simulink model "power_systerm_model"  (R2025b)
settings: Solver=FixedStepDiscrete  StartTime=0.0  StopTime=10.0  FixedStep=0.005  RelTol=1e-3
values from neighbouring files (symbols this model uses):
  motorMaxReactionTorque_Nm = 0.055562    [PowerSystemDict.sldd]
  motorMaxThrust_N = 4.17944622    [PowerSystemDict.sldd]
  motorTimeConstant_s = 0.005    [PowerSystemDict.sldd]
undefined symbols (not defined in the file or in its folder): motorArmLength_m, Thrust_Body, Torque_Body
settings Model: DataDictionary=PowerSystemDict.sldd  Creator=89447  LastModifiedBy=89447

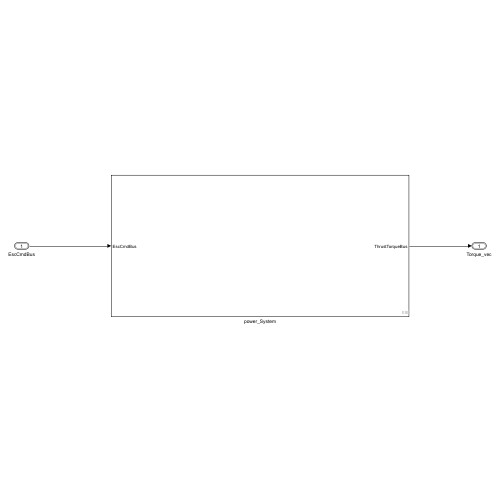
[thumbnail: Simulink's stored preview of the top-level diagram]
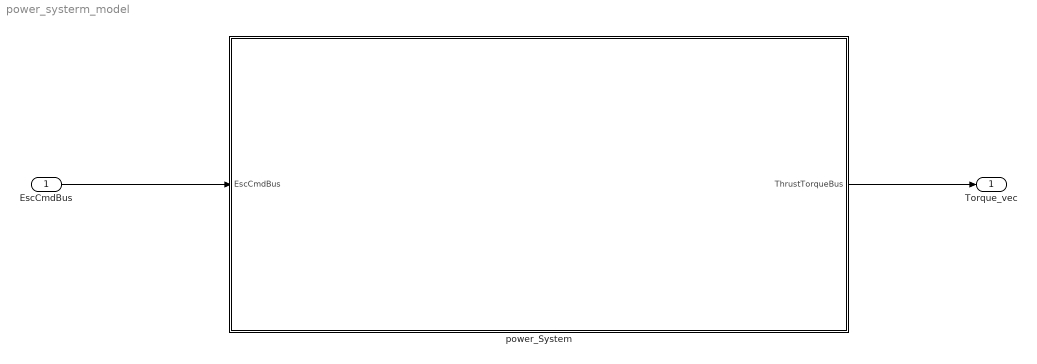
== system power_systerm_model ==
  EscCmdBus : Inport  OutDataTypeStr=Bus: EscCmdBus  LockScale=on  BusOutputAsStruct=on
  power_System : Subsystem
  Torque_vec : Outport  OutDataTypeStr=Bus: ThrustTorqueBus  LockScale=on  BusOutputAsStruct=on
  wires:
  EscCmdBus/1 -> power_System/1(EscCmdBus)
  power_System/1(ThrustTorqueBus) -> Torque_vec/1

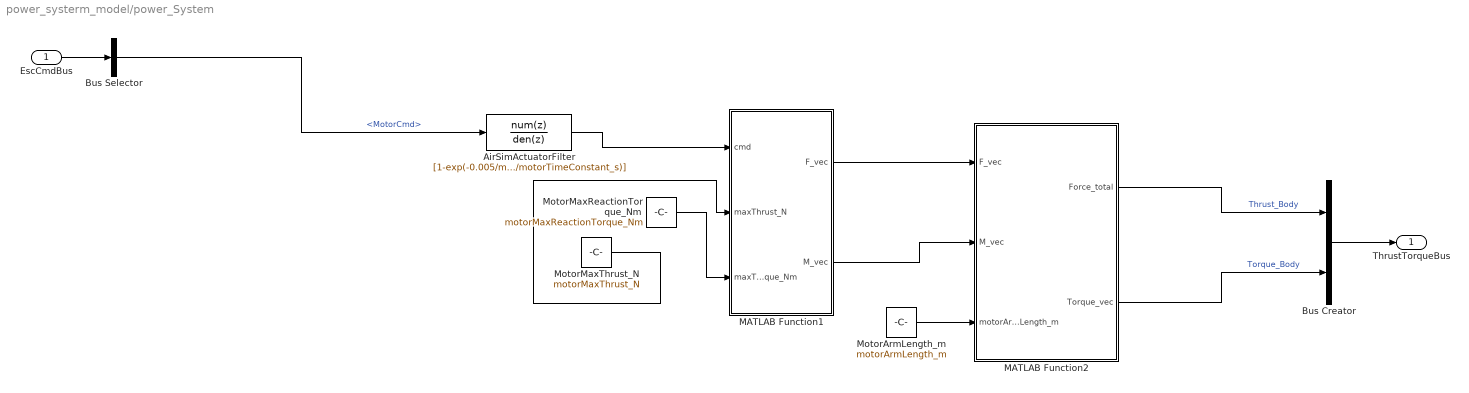
== system power_systerm_model/power_System ==
  EscCmdBus : Inport  OutDataTypeStr=Bus: EscCmdBus
  AirSimActuatorFilter : DiscreteTransferFcn  Numerator=[1-exp(-0.005/motorTimeConstant_s)]  Denominator=[1 -exp(-0.005/motorTimeConstant_s)]  SampleTime=0.005
  Bus Creator : BusCreator  Inputs=Thrust_Body,Torque_Body  OutDataTypeStr=Bus: ThrustTorqueBus
  Bus Selector : BusSelector  OutputSignals=MotorCmd
  MATLAB Function1 : MATLAB Function  TreatAsAtomicUnit=on
  MATLAB Function2 : MATLAB Function  TreatAsAtomicUnit=on
  MotorArmLength_m : Constant  Value=motorArmLength_m
  MotorMaxReactionTorque_Nm : Constant  Value=motorMaxReactionTorque_Nm
  MotorMaxThrust_N : Constant  Value=motorMaxThrust_N
  ThrustTorqueBus : Outport
  wires:
  MATLAB Function1/2(M_vec) -> MATLAB Function2/2(M_vec)
  MotorMaxReactionTorque_Nm/1 -> MATLAB Function1/3(maxTorque_Nm)
  MotorMaxThrust_N/1 -> MATLAB Function1/2(maxThrust_N)
  AirSimActuatorFilter/1 -> MATLAB Function1/1(cmd)
  MATLAB Function1/1(F_vec) -> MATLAB Function2/1(F_vec)
  MATLAB Function2/2(Torque_vec) -> Bus Creator/2  "Torque_Body"
  MotorArmLength_m/1 -> MATLAB Function2/3(motorArmLength_m)
  MATLAB Function2/1(Force_total) -> Bus Creator/1  "Thrust_Body"
  EscCmdBus/1 -> Bus Selector/1
  Bus Creator/1 -> ThrustTorqueBus/1
  Bus Selector/1 -> AirSimActuatorFilter/1  "<MotorCmd>"

== matlab function power_systerm_model/power_System/MATLAB Function1 ==
  data: cmd input; F_vec output; maxThrust_N input; maxTorque_Nm input; M_vec output
function [F_vec, M_vec] = fcn_airsim_rotors(cmd, maxThrust_N, maxTorque_Nm)
% AirSim RotorActuator: normalized command maps linearly to thrust and reaction torque.
cmd = max(single(0), min(single(1), single(cmd)));
F_vec = single(maxThrust_N) .* cmd;
M_vec = single(maxTorque_Nm) .* cmd;
end

== matlab function power_systerm_model/power_System/MATLAB Function2 ==
  data: F_vec input; Force_total output; M_vec input; motorArmLength_m input; Torque_vec output
function [Force_total, Torque_vec] = fcn_geometry_mixer(F_vec, M_vec, motorArmLength_m)
% AirSim QuadX rotor order and controller mixer sign convention.
k = single(sqrt(2)/2);
Force_total = single([0;0;sum(F_vec)]);
Tx = motorArmLength_m * k * (-F_vec(1) + F_vec(2) + F_vec(3) - F_vec(4));
Ty = motorArmLength_m * k * (-F_vec(1) + F_vec(2) - F_vec(3) + F_vec(4));
Tz = -M_vec(1) - M_vec(2) + M_vec(3) + M_vec(4);
Torque_vec = single([Tx; Ty; Tz]);
end
